simulink model "example_LoadFromFile"  (R2016b)
settings: Solver=VariableStepDiscrete  StartTime=0.0  StopTime=24*3600  RelTol=1e-3  EnableMultiTasking=on
libraries: carnot x2
settings Model: Creator=drhf  LastModifiedBy=drhf
settings DataIOCC: LimitDataPoints=on  SaveFormat=Array
settings OptimizationCC: ExpressionDepthLimit=2147483647  LifeSpan=inf
settings DebuggingCC: UnderspecifiedInitializationDetection=Classic  MergeDetectMultiDrivingBlocksExec=none  StateNameClashWarn=warning  SFUnexpectedBacktrackingDiag=warning  SFNoUnconditionalDefaultTransitionDiag=warning  SFExecutionAtInitializationDiag=none
settings HardwareCC: ProdBitPerPointer=32  ProdBitPerSizeT=32  ProdBitPerPtrDiffT=32  ProdLargestAtomicFloat=None  ProdIntDivRoundTo=Undefined  ProdEndianess=Unspecified  ProdWordSize=32  ProdHWDeviceType=32-bit Generic
settings ModelReferenceCC: PropagateSignalLabelsOutOfModel=off
settings GRTTargetCC: TargetLangStandard=C89/C90 (ANSI)  GeneratePreprocessorConditionals=Disable all  CombineOutputUpdateFcns=off  GRTInterface=on
settings ConfigComp: CovMetricSettings=dw  CovHtmlReporting=on  CovSaveCumulativeToWorkspaceVar=on  CovSaveSingleToWorkspaceVar=on  CovExternalEMLEnable=off

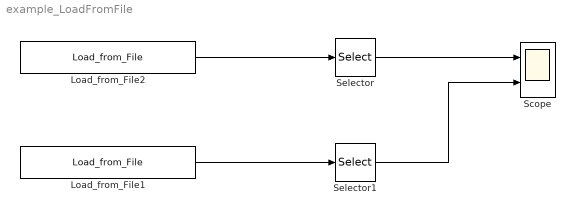
== system example_LoadFromFile ==
  Load_from_File1 : carnot/Load/General/Load_from_File  file=DE_TRY2010_07_averageYear  ext=.mat
  Load_from_File2 : carnot/Load/General/Load_from_File  file=DE_TRY2010_04_averageYear  ext=.mat
  Scope : Scope  NumInputPorts=2
  Selector : Selector  InputPortWidth=18  IndexOptions=Index vector (dialog)  Indices=[7]  OutputSizes=1
  Selector1 : Selector  InputPortWidth=18  IndexOptions=Index vector (dialog)  Indices=[7]  OutputSizes=1
  wires:
  Load_from_File2/1 -> Selector/1
  Selector/1 -> Scope/1
  Load_from_File1/1 -> Selector1/1
  Selector1/1 -> Scope/2
